simulink model "simulation_6dof"  (R2024b)
settings: Solver=VariableStepAuto  StartTime=0.0  StopTime=30  FixedStep=0.001  MaxStep=0.001  RelTol=1e-3
values from neighbouring files (symbols this model uses):
  g = 9.81    [params_environment.m]
  rho_air = 1.293    [params_environment.m]
  u_0 = 200    [params_environment.m]
undefined symbols (not defined in the file or in its folder): aero_length, c_aero, cp, mf
libraries: aerolibwind2 x2, aerolibanim x1, aerolibadyn x1, simulink x1, shared6dof x1, aerolibasang x1
settings Model: Creator=Finn  LastModifiedBy=finnb
settings RTWCC: GPUComputeCapability=3.5

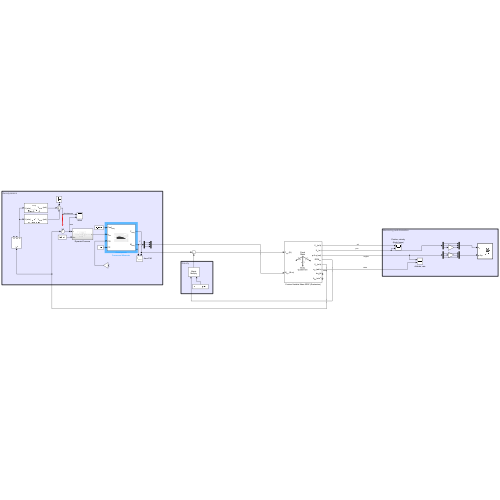
[thumbnail: Simulink's stored preview of the top-level diagram]
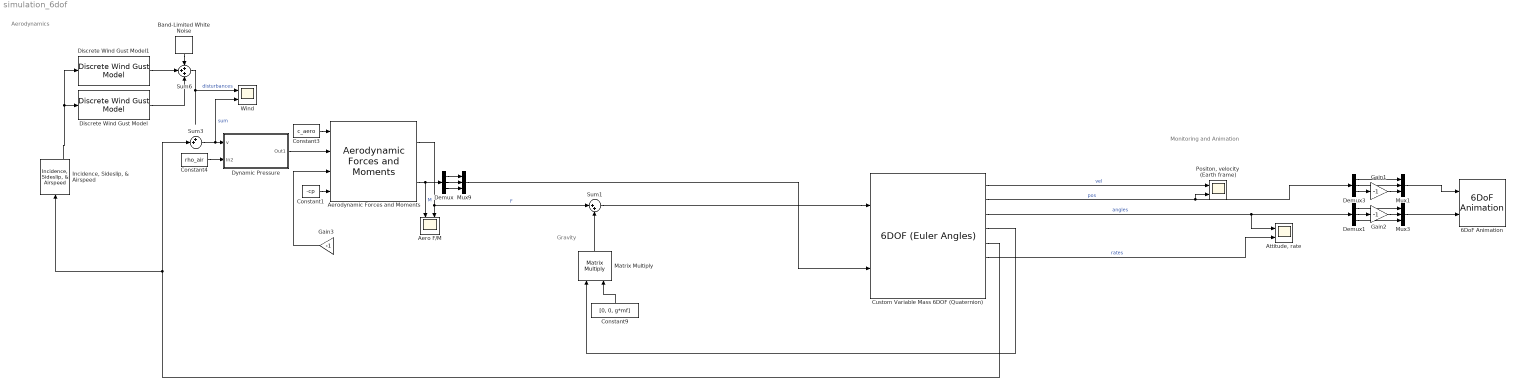
== system simulation_6dof ==
  note: Gravity
  note: Monitoring and Animation
  note: Aerodynamics
  6DoF Animation : aerolibanim/6DoF Animation  u1=[0 500 -10 10 -50 50]  u2=0.1  u3=2  u4=[-20 0 0]  u5=Fly alongside  u6=[0 100 30]  u7=10  u8=on
  Aero F/M : Scope  NumInputPorts=2
  "Aerodynamic Forces and Moments " : aerolibadyn/Aerodynamic Forces and Moments   inputAxes=Body  outputForceAxes=Body  outputMomentAxes=Body  S=aero_area_front  b=aero_length  cbar=aero_length
  "Attitude, rate" : Scope  NumInputPorts=2
  Band-Limited White Noise : simulink/Sources/Band-Limited White Noise  Cov=[1 2.5 1.5]  Ts=0.1  seed=[23970]
  Constant1 : Constant  Value=-cp
  Constant3 : Constant  Value=c_aero
  Constant4 : Constant  Value=rho_air
  Constant9 : Constant  Value=[0, 0, g*mf]
  Custom Variable Mass 6DOF (Quaternion) : shared6dof/6DOF (Euler Angles)  units=Metric (MKS)  mtype=Fixed  rep=Quaternion  xme_0=[0 0 0]  Vm_0=[-u_0, 0, 0]  eul_0=[0 90 0]  pm_0=[0 0 0]  mass_0=mf  mass_e=0.5  mass_f=2.0  inertia=Jf  inertia_e=eye(3)  inertia_f=2*eye(3)  k_quat=1.0  vre_flag=off  abi_flag=off  aMode=0  xme_statename=''  Vm_statename=''  eul_statename=''  quat_statename=''  pm_statename=''  mass_statename=''
      settings: LibrarySourceBlock=aerolib6dof2/Custom Variable Mass 6DOF (Quaternion)
  Demux : Demux  Outputs=3
  Demux1 : Demux  Outputs=3
  Demux3 : Demux  Outputs=3
  Discrete Wind Gust Model : aerolibwind2/Discrete Wind Gust Model  units=Metric (MKS)  Gx=on  Gy=on  Gz=on  t_0=1  d_m=[40 120 30]  v_m=[1.5 2.5 3.0]
  Discrete Wind Gust Model1 : aerolibwind2/Discrete Wind Gust Model  units=Metric (MKS)  Gx=on  Gy=on  Gz=on  t_0=2  d_m=[10 12 3]  v_m=[2 4 3]
  Dynamic Pressure : Subsystem
  Gain1 : Gain  Gain=-1
  Gain2 : Gain  Gain=-1
  Gain3 : Gain  Gain=-1
  "Incidence, Sideslip, & Airspeed" : aerolibasang/Incidence, Sideslip, & Airspeed
  Matrix Multiply : Product  Multiplication=Matrix(*)
  Mux1 : Mux  Inputs=3
  Mux3 : Mux  Inputs=3
  Mux9 : Mux  Inputs=3
  "Positon, velocity (Earth frame)" : Scope  NumInputPorts=2
  Sum1 : Sum  Inputs=|++
  Sum3 : Sum  Inputs=++|
  Sum6 : Sum  Inputs=+++
  Wind : Scope  NumInputPorts=2
  wires:
  Custom Variable Mass 6DOF (Quaternion)/2 -> "Positon, velocity (Earth frame)"/2, Demux3/1  "pos"
  Constant1/1 -> "Aerodynamic Forces and Moments "/4
  Constant3/1 -> "Aerodynamic Forces and Moments "/1
  Custom Variable Mass 6DOF (Quaternion)/6 -> "Attitude, rate"/2  "rates"
  "Aerodynamic Forces and Moments "/2 -> Aero F/M/1, Demux/1  "M"
  Demux3/1 -> Mux1/1
  Mux1/1 -> 6DoF Animation/1
  Demux3/2 -> Mux1/2
  Dynamic Pressure/1(Out1) -> "Aerodynamic Forces and Moments "/2
  Constant4/1 -> Dynamic Pressure/2(In2)
  Sum3/1 -> Wind/2, Dynamic Pressure/1(v)  "sum"
  Sum6/1 -> Wind/1  "disturbances"
  Discrete Wind Gust Model/1 -> Sum6/3
  "Aerodynamic Forces and Moments "/1 -> Aero F/M/2, Sum1/1  "F"
  Sum1/1 -> Custom Variable Mass 6DOF (Quaternion)/1
  Band-Limited White Noise/1 -> Sum6/1
  Discrete Wind Gust Model1/1 -> Sum6/2
  Demux/3 -> Mux9/3
  Demux/2 -> Mux9/2
  Custom Variable Mass 6DOF (Quaternion)/5 -> Sum3/2, "Incidence, Sideslip, & Airspeed"/1
  Demux1/1 -> Mux3/1
  Gain2/1 -> Mux3/2
  Demux1/3 -> Mux3/3
  Mux3/1 -> 6DoF Animation/2
  Demux3/3 -> Gain1/1
  Custom Variable Mass 6DOF (Quaternion)/3 -> Demux1/1, "Attitude, rate"/1  "angles"
  "Incidence, Sideslip, & Airspeed"/3 -> Discrete Wind Gust Model1/1, Discrete Wind Gust Model/1
  Gain1/1 -> Mux1/3
  Matrix Multiply/1 -> Sum1/2
  Custom Variable Mass 6DOF (Quaternion)/4 -> Matrix Multiply/1
  Constant9/1 -> Matrix Multiply/2
  Demux1/2 -> Gain2/1
  Mux9/1 -> Custom Variable Mass 6DOF (Quaternion)/2
  Gain3/1 -> "Aerodynamic Forces and Moments "/3
  Demux/1 -> Mux9/1
  Custom Variable Mass 6DOF (Quaternion)/1 -> "Positon, velocity (Earth frame)"/1  "vel"

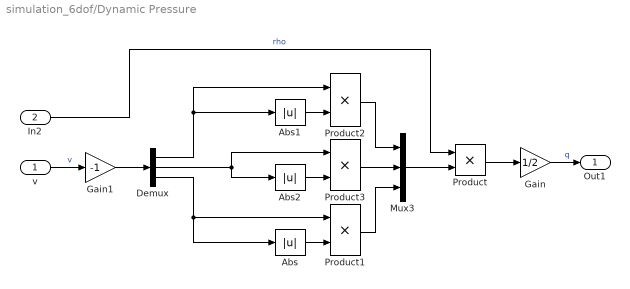
== system simulation_6dof/Dynamic Pressure ==
  v : Inport
  In2 : Inport  Port=2
  Abs : Abs  SaturateOnIntegerOverflow=off
  Abs1 : Abs  SaturateOnIntegerOverflow=off
  Abs2 : Abs  SaturateOnIntegerOverflow=off
  Demux : Demux  Outputs=3
  Gain : Gain  Gain=1/2
  Gain1 : Gain  Gain=-1
  Mux3 : Mux  Inputs=3
  Product{,1..3} (4 alike) : Product
  Out1 : Outport
  wires:
  Product1/1 -> Mux3/3
  Abs1/1 -> Product2/2
  Product2/1 -> Mux3/1
  Abs/1 -> Product1/2
  v/1 -> Gain1/1  "v"
  Abs2/1 -> Product3/2
  Product3/1 -> Mux3/2
  In2/1 -> Product/1  "rho"
  Gain/1 -> Out1/1  "q"
  Mux3/1 -> Product/2
  Product/1 -> Gain/1
  Demux/1 -> Product2/1, Abs1/1
  Demux/2 -> Abs2/1, Product3/1
  Demux/3 -> Abs/1, Product1/1
  Gain1/1 -> Demux/1
